simulink model "P3_10_1"  (R2024b)
settings: Solver=VariableStepAuto  StartTime=0.0  StopTime=10.0  RelTol=1e-3
values from neighbouring files (symbols this model uses):
  th = 60    [P3_10.m]
  wn = sqrt(2)    [P3_10.m]
  x = sqrt(abs(1 - z^2))    [P3_10.m]
  y0 = 0.5    [P3_10.m]
  z = 1/sqrt(2)    [P3_10.m]    (also in P_4.m = [.1 .2 .4 .7 1 2])
settings Model: Creator=Rj Avro Biswas  LastModifiedBy=Rj Avro Biswas

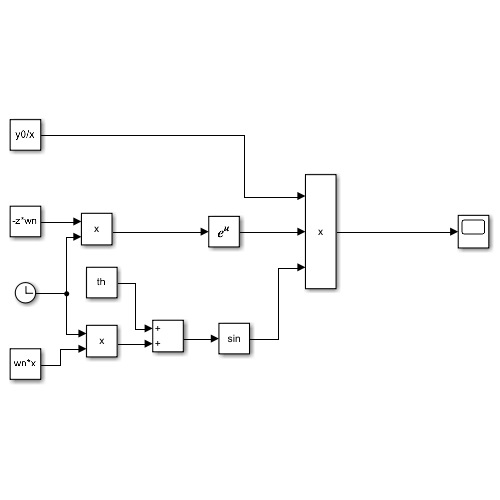
[thumbnail: Simulink's stored preview of the top-level diagram]
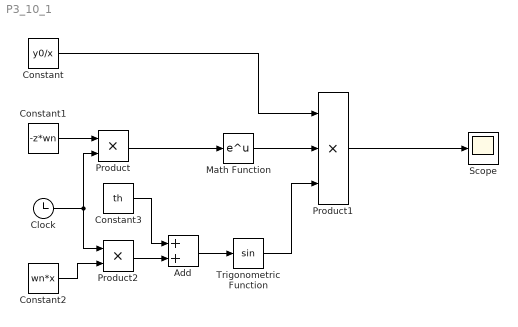
== system P3_10_1 ==
  Add : Sum
  Clock : Clock
  Constant : Constant  Value=y0/x
  Constant1 : Constant  Value=-z*wn
  Constant2 : Constant  Value=wn*x
  Constant3 : Constant  Value=th
  Math Function : Math
  Product : Product
  Product1 : Product  Inputs=3
  Product2 : Product
  Scope : Scope
  Trigonometric Function : Trigonometry
  wires:
  Product/1 -> Math Function/1
  Constant/1 -> Product1/1
  Math Function/1 -> Product1/2
  Product1/1 -> Scope/1
  Trigonometric Function/1 -> Product1/3
  Constant1/1 -> Product/1
  Clock/1 -> Product2/1, Product/2
  Constant2/1 -> Product2/2
  Add/1 -> Trigonometric Function/1
  Product2/1 -> Add/2
  Constant3/1 -> Add/1
